simulink model "SF012A_HysCmp"  (R2013b)
settings: Solver=FixedStepDiscrete  StartTime=0.0  StopTime=1  FixedStep=.002  RelTol=1e-3
values from neighbouring files (symbols this model uses):
  ARCHGLBPRM_2MILLISEC_SEC_F32 = DataDict.Constant    [SF012A_HysCmp_DataDict.m]
  EPSILON_ULS_F32 = DataDict.Constant    [SF012A_HysCmp_DataDict.m]
  FLTINJ_HYSCMP_HYSCMPCMD = DataDict.Constant    [SF012A_HysCmp_DataDict.m]
  HysCmpAssiInpLim = DataDict.Calibration    [SF012A_HysCmp_DataDict.m]
  HysCmpOutpLim = DataDict.Calibration    [SF012A_HysCmp_DataDict.m]
  HysCmpRevGain = DataDict.Calibration    [SF012A_HysCmp_DataDict.m]
  HysCmpRiseX = DataDict.Calibration    [SF012A_HysCmp_DataDict.m]
  HysCmpRiseY = DataDict.Calibration    [SF012A_HysCmp_DataDict.m]
  HYSRISEYLIM_ULS_F32 = DataDict.Constant    [SF012A_HysCmp_DataDict.m]
  HYSSATNLOWLIM_HWNWTMTR_F32 = DataDict.Constant    [SF012A_HysCmp_DataDict.m]
  SysGlbPrmSysTqRat = DataDict.ImprtdCal    [SF012A_HysCmp_DataDict.m]
libraries: FixdToFloat x18, FloatToFixd x14, LnrIntrpn x12, NxtrAbslt x10, NxtrLim x8, Fil x6, NxtrSign x5, simulink x2, NxtrMath x1, BilnrIntrpnMplX x1, NxtrMax x1
(part 3 of 3)

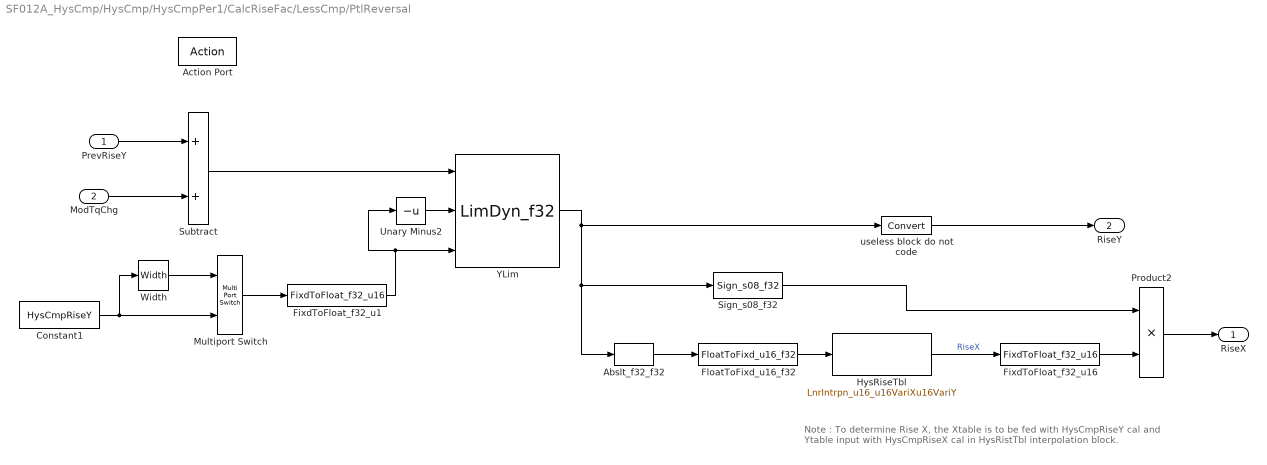
== system SF012A_HysCmp/HysCmp/HysCmpPer1/CalcRiseFac/LessCmp/PtlReversal ==
  note: Note : To determine Rise X, the Xtable is to be fed with HysCmpRiseY cal
      | and Ytable input with HysCmpRiseX cal in HysRistTbl interpolation block.
  PrevRiseY : Inport  RequirementInfo={'linktype_rmi_doors' '0000a52c (/E-STEER Core/SubSystem Specifications/Application Functions/SF012A Hysteresis Compensation)' '#SF012A_430' 'true' 'REQ:SF012A_430' '' } %GIDa_ae377267_69ba_4941_9cf5_410eee12eaba
  ModTqChg : Inport  RequirementInfo={'linktype_rmi_doors' '0000a52c (/E-STEER Core/SubSystem Specifications/Application Functions/SF012A Hysteresis Compensation)' '#SF012A_430' 'true' 'REQ:SF012A_430' '' } %GIDa_6760b101_0e15_4759_a6ad_05ae0b9af739  Port=2
  Action Port : ActionPort  ActionType=then
  Abslt_f32_f32 : NxtrAbslt/Abslt_f32_f32  RequirementInfo={'linktype_rmi_doors' '0000a52c (/E-STEER Core/SubSystem Specifications/Application Functions/SF012A Hysteresis Compensation)' '#SF012A_432' 'true' 'REQ:SF012A_432' '' } %GIDa_00f04870_9655_4842_9346_d909c5ec5998  SFunctionSpec=single y1 = Abslt_f32_f32(single u1)
      settings: AttributesFormatString=%<Name>
  Constant1 : Constant  RequirementInfo={'linktype_rmi_doors' '0000a52c (/E-STEER Core/SubSystem Specifications/Application Functions/SF012A Hysteresis Compensation)' '#SF012A_431' 'true' 'REQ:SF012A_431' '' } %GIDa_c15f61e3_26bc_40b7_a2fe_dcbf6169f9a0  Value=HysCmpRiseY
  FixdToFloat_f32_u1 : FixdToFloat/FixdToFloat_f32_u16  RequirementInfo={'linktype_rmi_doors' '0000a52c (/E-STEER Core/SubSystem Specifications/Application Functions/SF012A Hysteresis Compensation)' '#SF012A_431' 'true' 'REQ:SF012A_431' '' } %GIDa_25b173c8_7a8c_4d0c_9fc4_53956c72abd8  Param1=14
  FixdToFloat_f32_u16 : FixdToFloat/FixdToFloat_f32_u16  RequirementInfo={'linktype_rmi_doors' '0000a52c (/E-STEER Core/SubSystem Specifications/Application Functions/SF012A Hysteresis Compensation)' '#SF012A_432' 'true' 'REQ:SF012A_432' '' } %GIDa_1372204b_5231_4d84_934b_b04151b092ad  Param1=14
  FloatToFixd_u16_f32 : FloatToFixd/FloatToFixd_u16_f32  RequirementInfo={'linktype_rmi_doors' '0000a52c (/E-STEER Core/SubSystem Specifications/Application Functions/SF012A Hysteresis Compensation)' '#SF012A_432' 'true' 'REQ:SF012A_432' '' } %GIDa_0ba03c1b_58b7_483b_86c2_6e90989f9fd1  Param1=14
  HysRiseTbl : LnrIntrpn/LnrIntrpn_u16_u16VariXu16VariY  RequirementInfo={'linktype_rmi_doors' '0000a52c (/E-STEER Core/SubSystem Specifications/Application Functions/SF012A Hysteresis Compensation)' '#SF012A_432' 'true' 'REQ:SF012A_432' '' } %GIDa_b688975c_0fca_4d24_9c5a_707fbdb216fd  XTbl=HysCmpRiseY  YTbl=HysCmpRiseX
      settings: AttributesFormatString=Lnr ( u16VariX , u16VariY )
  Multiport Switch : MultiPortSwitch  RequirementInfo={'linktype_rmi_doors' '0000a52c (/E-STEER Core/SubSystem Specifications/Application Functions/SF012A Hysteresis Compensation)' '#SF012A_431' 'true' 'REQ:SF012A_431' '' } %GIDa_b0d84669_019e_49f7_88fd_91fb0ead013b  Inputs=1
  Product2 : Product  RequirementInfo={'linktype_rmi_doors' '0000a52c (/E-STEER Core/SubSystem Specifications/Application Functions/SF012A Hysteresis Compensation)' '#SF012A_432' 'true' 'REQ:SF012A_432' '' } %GIDa_1261776e_4b62_4b28_99c9_cb7ac2379d34  RndMeth=Zero
  Sign_s08_f32 : NxtrSign/Sign_s08_f32  RequirementInfo={'linktype_rmi_doors' '0000a52c (/E-STEER Core/SubSystem Specifications/Application Functions/SF012A Hysteresis Compensation)' '#SF012A_432' 'true' 'REQ:SF012A_432' '' } %GIDa_4466eb62_f4cc_43ac_943e_763609f9e5e6  SFunctionSpec=int8 y1 = Sign_s08_f32(single u1)
  Subtract : Sum  RequirementInfo={'linktype_rmi_doors' '0000a52c (/E-STEER Core/SubSystem Specifications/Application Functions/SF012A Hysteresis Compensation)' '#SF012A_430' 'true' 'REQ:SF012A_430' '' } %GIDa_cf9ca45a_936d_4c0a_9e0a_bfcc6b1790af  RndMeth=Zero
  Unary Minus2 : UnaryMinus  RequirementInfo={'linktype_rmi_doors' '0000a52c (/E-STEER Core/SubSystem Specifications/Application Functions/SF012A Hysteresis Compensation)' '#SF012A_431' 'true' 'REQ:SF012A_431' '' } %GIDa_352db724_20c7_4cd1_b141_4e08960d1a84
  Width : Width  RequirementInfo={'linktype_rmi_doors' '0000a52c (/E-STEER Core/SubSystem Specifications/Application Functions/SF012A Hysteresis Compensation)' '#SF012A_431' 'true' 'REQ:SF012A_431' '' } %GIDa_4dbc85cc_9279_49c5_81ef_8aebbdbf85d7  DataType=uint16
  YLim : NxtrLim/LimDyn_f32  RequirementInfo={'linktype_rmi_doors' '0000a52c (/E-STEER Core/SubSystem Specifications/Application Functions/SF012A Hysteresis Compensation)' '#SF012A_431' 'true' 'REQ:SF012A_431' '' } %GIDa_ea0149ef_873d_4954_a8cd_f86f4057953c
  useless block do not code : DataTypeConversion  RequirementInfo={'linktype_rmi_doors' '0000a52c (/E-STEER Core/SubSystem Specifications/Application Functions/SF012A Hysteresis Compensation)' '#SF012A_432' 'true' 'REQ:SF012A_432' '' } %GIDa_d3ae2879_f1b0_4498_9690_7393a8bd8e48
  RiseX : Outport  RequirementInfo={'linktype_rmi_doors' '0000a52c (/E-STEER Core/SubSystem Specifications/Application Functions/SF012A Hysteresis Compensation)' '#SF012A_432' 'true' 'REQ:SF012A_432' '' } %GIDa_78a4e6f6_6d3b_4bfa_a6e3_0964dc3046a9
  RiseY : Outport  Port=2
  wires:
  PrevRiseY/1 -> Subtract/1
  ModTqChg/1 -> Subtract/2
  Subtract/1 -> YLim/1
  Unary Minus2/1 -> YLim/2
  YLim/1 -> Abslt_f32_f32/1, Sign_s08_f32/1, useless block do not code/1
  HysRiseTbl/1 -> FixdToFloat_f32_u16/1  "RiseX"
  Abslt_f32_f32/1 -> FloatToFixd_u16_f32/1
  Sign_s08_f32/1 -> Product2/1
  FloatToFixd_u16_f32/1 -> HysRiseTbl/1
  Product2/1 -> RiseX/1
  FixdToFloat_f32_u16/1 -> Product2/2
  Constant1/1 -> Multiport Switch/2, Width/1
  Width/1 -> Multiport Switch/1
  Multiport Switch/1 -> FixdToFloat_f32_u1/1
  FixdToFloat_f32_u1/1 -> Unary Minus2/1, YLim/3
  useless block do not code/1 -> RiseY/1

== system SF012A_HysCmp/HysCmp/HysCmpPer1/CalcRiseFac/MoreCmp/CopyRight2 ==

== system SF012A_HysCmp/HysCmp/HysCmpPer1/CalcRiseFac/NoChg/CopyRight2 ==

== system SF012A_HysCmp/HysCmp/HysCmpPer1/FilAndLimInp/If Action Subsystem/CopyRight2 ==

== system SF012A_HysCmp/HysCmp/HysCmpPer1/FilAndLimInp/If Action Subsystem1/CopyRight2 ==

== system SF012A_HysCmp/HysCmp/HysCmpPer1/FilHysCmpOutp/HysCmp/CopyRight2 ==

== system SF012A_HysCmp/HysCmp/HysCmpPer1/FilHysCmpOutp/Zero_Command/CopyRight2 ==
